simulink model "out_stage_test"  (R2020a)
settings: Solver=VariableStepAuto  StartTime=0.0  StopTime=0.025  RelTol=1e-3
undefined symbols (not defined in the file): debouncer_cycles, FPGA_CLK, FPGA_Ts, MECOS_CTRLR_Ts, PHCTRLR_CLK
libraries: xbsIndex_r4 x55, simulink x1
settings Model: Creator=valbas  LastModifiedBy=valbas

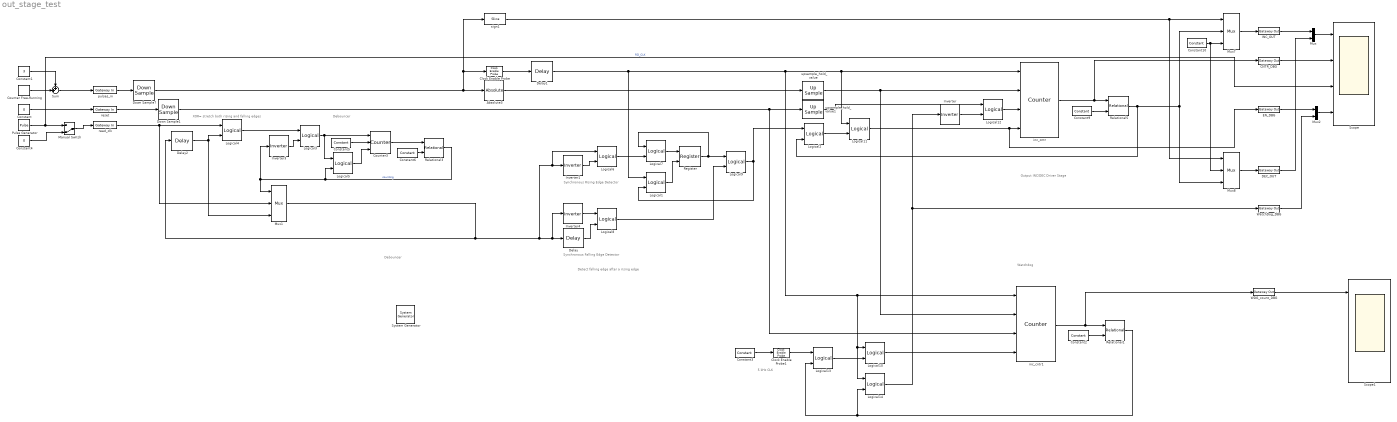
== system out_stage_test ==
  note: Output INC/DEC Driver Stage
  note: XOR= stretch both rising and falling edges
  note: Debouncer
  note: Synchronous Rising Edge Detector
  note: Synchronous Falling Edge Detector
  note: Debouncer
  note: Detect falling edge after a rising edge
  note: Watchdog
  note: 5 kHz CLK
  " System Generator" : xbsIndex_r4/ System Generator  Tag=genX  xilinxfamily=zynquplus  part=xczu7ev  speed=-2-e  package=ffvc1156  synthesis_tool=Vivado  clock_wrapper=Clock Enables  directory=./netlist  proj_type=Vivado  Synth_file=Vivado Synthesis Defaults  Impl_file=Vivado Implementation Defaults  testbench=off  simulink_period=FPGA_Ts  sysclk_period=FPGA_Ts*1e9  dcm_input_clock_period=10  incr_netlist=off  trim_vbits=Everywhere in SubSystem  dbl_ovrd=According to Block Masks  core_generation=According to Block Masks  run_coregen=off  deprecated_control=off  eval_field=0  block_type=sysgen
  Absolute3 : xbsIndex_r4/Absolute  precision=User Defined  arith_type="Signed  (2's comp)"  n_bits=22  bin_pt=0  quantization=Truncate  overflow=Wrap  en=off  latency=0  dbl_ovrd=off  block_type=abs
  CNTR_DBG : xbsIndex_r4/Gateway Out  inherit_from_input=on  hdl_port=on  rows=1  columns=1  UseAsDAC=off  DACChannel='1'  interface=None  automatic_assignment=on  address_offset=hex2dec('00')  intf_name=''  intf_description=''  timing_constraint=None  locs_specified=off  LOCs={}  io_standard={}  block_type=gatewayout
  Clock Enable Probe : xbsIndex_r4/Clock Enable Probe  inherit_constraints=on  block_type=ceprobe
      settings: infoedit="Clock enable extractor.  Produces a Boolean output that mirrors the hardware clock enable associated with the input sample rate.<br><br>Hardware notes: in hardware this block costs nothing."
  Clock Enable Probe1 : xbsIndex_r4/Clock Enable Probe  inherit_constraints=on  block_type=ceprobe
      settings: infoedit="Clock enable extractor.  Produces a Boolean output that mirrors the hardware clock enable associated with the input sample rate.<br><br>Hardware notes: in hardware this block costs nothing."
  Constant : Constant  Value=0
  Constant1 : Constant  Value=3
  Constant10 : xbsIndex_r4/Constant  const=0  gui_display_data_type=Boolean  arith_type=Boolean  n_bits=22  bin_pt=0  preci_type=Single  exp_width=8  frac_width=24  explicit_period=off  period=1  equ=P=C  opselect=C  inp2=PCIN>>17  opr=+  inp1=P  carry=CIN  dbl_ovrd=off  block_type=constant
  Constant2 : xbsIndex_r4/Constant  const=0  gui_display_data_type=Fixed-point  arith_type=Signed (2's comp)  n_bits=22  bin_pt=0  preci_type=Single  exp_width=8  frac_width=24  explicit_period=off  period=1  equ=P=C  opselect=C  inp2=PCIN>>17  opr=+  inp1=P  carry=CIN  dbl_ovrd=off  block_type=constant
  Constant3 : xbsIndex_r4/Constant  const=1  gui_display_data_type=Boolean  arith_type=Boolean  n_bits=7  bin_pt=0  preci_type=Single  exp_width=8  frac_width=24  explicit_period=on  period=PWM_Ts  equ=P=C  opselect=C  inp2=PCIN>>17  opr=+  inp1=P  carry=CIN  dbl_ovrd=off  block_type=constant
  Constant4 : Constant  Value=0
  Constant5 : xbsIndex_r4/Constant  const=debouncer_cycles  gui_display_data_type=Fixed-point  arith_type=Unsigned  n_bits=7  bin_pt=0  preci_type=Single  exp_width=8  frac_width=24  explicit_period=off  period=1  equ=P=C  opselect=C  inp2=PCIN>>17  opr=+  inp1=P  carry=CIN  dbl_ovrd=off  block_type=constant
  Constant6 : xbsIndex_r4/Constant  const=1  gui_display_data_type=Fixed-point  arith_type=Unsigned  n_bits=7  bin_pt=0  preci_type=Single  exp_width=8  frac_width=24  explicit_period=off  period=1  equ=P=C  opselect=C  inp2=PCIN>>17  opr=+  inp1=P  carry=CIN  dbl_ovrd=off  block_type=constant
  Constant9 : xbsIndex_r4/Constant  const=0  gui_display_data_type=Fixed-point  arith_type=Signed (2's comp)  n_bits=22  bin_pt=0  preci_type=Single  exp_width=8  frac_width=24  explicit_period=off  period=1  equ=P=C  opselect=C  inp2=PCIN>>17  opr=+  inp1=P  carry=CIN  dbl_ovrd=off  block_type=constant
  Counter Free-Running : simulink/Sources/Counter Free-Running  NumBits=4  tsamp=PHCTRLR_Ts
  Counter3 : xbsIndex_r4/Counter  cnt_type=Free Running  cnt_to=2  operation=Down  start_count=1  cnt_by_val=1  arith_type=Unsigned  n_bits=7  bin_pt=0  load_pin=on  rst=off  en=on  explicit_period=on  period=FPGA_Ts  use_behavioral_HDL=off  implementation=Fabric  dbl_ovrd=off  block_type=counter
  DEC_OUT : xbsIndex_r4/Gateway Out  inherit_from_input=on  hdl_port=on  rows=1  columns=1  UseAsDAC=off  DACChannel='1'  interface=None  automatic_assignment=on  address_offset=hex2dec('00')  intf_name=''  intf_description=''  timing_constraint=None  locs_specified=off  LOCs={}  io_standard={}  block_type=gatewayout
  Delay : xbsIndex_r4/Delay  rst=off  infoeditControl=Selection of Reset will increase slice count due to use of real FFs and instead of SRLs  en=off  latency=1  reg_retiming=off  dbl_ovrd=off  block_type=delay
  Delay1 : xbsIndex_r4/Delay  rst=off  infoeditControl=Selection of Reset will increase slice count due to use of real FFs and instead of SRLs  en=off  latency=1  reg_retiming=off  dbl_ovrd=off  block_type=delay
  Delay2 : xbsIndex_r4/Delay  rst=off  infoeditControl=Selection of Reset will increase slice count due to use of real FFs and instead of SRLs  en=off  latency=1  reg_retiming=off  dbl_ovrd=off  block_type=delay
  Down Sample1 : xbsIndex_r4/Down Sample  sample_ratio=FPGA_CLK/PHCTRLR_CLK  sample_phase="Last Value of Frame  (most efficient)"  en=off  rst=off  latency=1  dbl_ovrd=off  block_type=dsamp
  Down Sample7 : xbsIndex_r4/Down Sample  sample_ratio=FPGA_CLK/PHCTRLR_CLK  sample_phase="Last Value of Frame  (most efficient)"  en=off  rst=off  latency=1  dbl_ovrd=off  block_type=dsamp
  EN_DBG : xbsIndex_r4/Gateway Out  inherit_from_input=on  hdl_port=on  rows=1  columns=1  UseAsDAC=off  DACChannel='1'  interface=None  automatic_assignment=on  address_offset=hex2dec('00')  intf_name=''  intf_description=''  timing_constraint=None  locs_specified=off  LOCs={}  io_standard={}  block_type=gatewayout
  INC_OUT : xbsIndex_r4/Gateway Out  inherit_from_input=on  hdl_port=on  rows=1  columns=1  UseAsDAC=off  DACChannel='1'  interface=None  automatic_assignment=on  address_offset=hex2dec('00')  intf_name=''  intf_description=''  timing_constraint=None  locs_specified=off  LOCs={}  io_standard={}  block_type=gatewayout
  Inverter : xbsIndex_r4/Inverter  en=off  latency=0  dbl_ovrd=off  block_type=inv
  Inverter1 : xbsIndex_r4/Inverter  en=off  latency=1  dbl_ovrd=off  block_type=inv
  Inverter3 : xbsIndex_r4/Inverter  en=off  latency=0  dbl_ovrd=off  block_type=inv
  Inverter4 : xbsIndex_r4/Inverter  en=off  latency=0  dbl_ovrd=off  block_type=inv
  Logical{1,5,7,10..12,14} (7 alike) : xbsIndex_r4/Logical  logical_function=OR  inputs=2  en=off  latency=0  precision=Full  arith_type=Unsigned  n_bits=16  bin_pt=0  align_bp=on  dbl_ovrd=off  block_type=logical
  Logical{2..3,6,8..9,13} (6 alike) : xbsIndex_r4/Logical  logical_function=AND  inputs=2  en=off  latency=0  precision=Full  arith_type=Unsigned  n_bits=16  bin_pt=0  align_bp=on  dbl_ovrd=off  block_type=logical
  Logical4 : xbsIndex_r4/Logical  logical_function=XOR  inputs=2  en=off  latency=0  precision=Full  arith_type=Unsigned  n_bits=16  bin_pt=0  align_bp=on  dbl_ovrd=off  block_type=logical
  Manual Switch : ManualSwitch  CurrentSetting=0
  Mux : Mux  Inputs=2
  Mux1 : xbsIndex_r4/Mux  inputs=2  en=off  latency=0  precision=Full  arith_type=Unsigned  n_bits=16  bin_pt=14  quantization=Truncate  overflow=Wrap  dbl_ovrd=off  block_type=mux
  Mux2 : Mux  Inputs=2
  Mux7 : xbsIndex_r4/Mux  inputs=2  en=off  latency=0  precision=Full  arith_type=Unsigned  n_bits=16  bin_pt=14  quantization=Truncate  overflow=Wrap  dbl_ovrd=off  block_type=mux
  Mux8 : xbsIndex_r4/Mux  inputs=2  en=off  latency=0  precision=Full  arith_type=Unsigned  n_bits=16  bin_pt=14  quantization=Truncate  overflow=Wrap  dbl_ovrd=off  block_type=mux
  Pulse Generator : DiscretePulseGenerator  PulseType=Time based  Period=MECOS_CTRLR_Ts  PulseWidth=50
  Register : xbsIndex_r4/Register  init=0  rst=on  en=off  dbl_ovrd=off  block_type=register
  Relational1 : xbsIndex_r4/Relational  mode=a!=b  op_type=Bool  en=off  latency=0  dbl_ovrd=off  block_type=relational
  Relational3 : xbsIndex_r4/Relational  mode=a!=b  op_type=Bool  en=off  latency=0  dbl_ovrd=off  block_type=relational
  Relational5 : xbsIndex_r4/Relational  mode=a!=b  op_type=Bool  en=off  latency=0  dbl_ovrd=off  block_type=relational
  Scope : Scope  NumInputPorts=4
  Scope1 : Scope  NumInputPorts=4
  Sum : Sum  Inputs=++|
  WDG_count_DBG : xbsIndex_r4/Gateway Out  inherit_from_input=on  hdl_port=on  rows=1  columns=1  UseAsDAC=off  DACChannel='1'  interface=None  automatic_assignment=on  address_offset=hex2dec('00')  intf_name=''  intf_description=''  timing_constraint=None  locs_specified=off  LOCs={}  io_standard={}  block_type=gatewayout
  WatchDog_DBG : xbsIndex_r4/Gateway Out  inherit_from_input=on  hdl_port=on  rows=1  columns=1  UseAsDAC=off  DACChannel='1'  interface=None  automatic_assignment=on  address_offset=hex2dec('00')  intf_name=''  intf_description=''  timing_constraint=None  locs_specified=off  LOCs={}  io_standard={}  block_type=gatewayout
  inc_cntr : xbsIndex_r4/Counter  cnt_type=Free Running  cnt_to=0  operation=Down  start_count=0  cnt_by_val=1  arith_type="Signed  (2's comp)"  n_bits=22  bin_pt=0  load_pin=on  rst=on  en=on  explicit_period=on  period=FPGA_Ts  use_behavioral_HDL=off  implementation=DSP48  dbl_ovrd=off  block_type=counter
  inc_cntr1 : xbsIndex_r4/Counter  cnt_type=Free Running  cnt_to=0  operation=Down  start_count=0  cnt_by_val=1  arith_type="Signed  (2's comp)"  n_bits=22  bin_pt=0  load_pin=on  rst=on  en=on  explicit_period=on  period=FPGA_Ts  use_behavioral_HDL=off  implementation=DSP48  dbl_ovrd=off  block_type=counter
  pulses_in : xbsIndex_r4/Gateway In  gui_display_data_type=Fixed-point  arith_type="Signed  (2's comp)"  n_bits=22  bin_pt=0  preci_type=Single  exp_width=8  frac_width=24  rows=1  columns=1  quantization="Round  (unbiased: +/- Inf)"  overflow=Saturate  period=FPGA_Ts  UseAsADC=off  ADCChannel='1'  interface=None  automatic_assignment=on  address_offset=hex2dec('00')  intf_name=''  intf_description=''  default_value=0  timing_constraint=None  locs_specified=off  LOCs={}  io_standard={}  inherit_from_input=off  hdl_port=on  dbl_ovrd=off  block_type=gatewayin
  read_clk : xbsIndex_r4/Gateway In  gui_display_data_type=Boolean  arith_type=Boolean  n_bits=16  bin_pt=14  preci_type=Single  exp_width=8  frac_width=24  rows=1  columns=1  quantization="Round  (unbiased: +/- Inf)"  overflow=Saturate  period=FPGA_Ts  UseAsADC=off  ADCChannel='1'  interface=None  automatic_assignment=on  address_offset=hex2dec('00')  intf_name=''  intf_description=''  default_value=0  timing_constraint=None  locs_specified=off  LOCs={}  io_standard={}  inherit_from_input=off  hdl_port=on  dbl_ovrd=off  block_type=gatewayin
  reset : xbsIndex_r4/Gateway In  gui_display_data_type=Boolean  arith_type=Boolean  n_bits=16  bin_pt=14  preci_type=Single  exp_width=8  frac_width=24  rows=1  columns=1  quantization="Round  (unbiased: +/- Inf)"  overflow=Saturate  period=FPGA_Ts  UseAsADC=off  ADCChannel='1'  interface=None  automatic_assignment=on  address_offset=hex2dec('00')  intf_name=''  intf_description=''  default_value=0  timing_constraint=None  locs_specified=off  LOCs={}  io_standard={}  inherit_from_input=off  hdl_port=on  dbl_ovrd=off  block_type=gatewayin
  sign1 : xbsIndex_r4/Slice  nbits=1  boolean_output=on  mode=Upper Bit Location + Width  bit1=0  base1=MSB of Input  bit0=0  base0=LSB of Input  dbl_ovrd=off  block_type=slice
  upsample_hold_value : xbsIndex_r4/Up Sample  sample_ratio=FPGA_CLK/PHCTRLR_CLK  copy_samples=on  en=off  latency=0  dbl_ovrd=off  block_type=usamp
  upsample_hold_value1 : xbsIndex_r4/Up Sample  sample_ratio=FPGA_CLK/PHCTRLR_CLK  copy_samples=on  en=off  latency=0  dbl_ovrd=off  block_type=usamp
  wires:
  Delay1/1 -> Logical1/1, Logical14/1, Logical10/1, inc_cntr1/1, inc_cntr/1, Logical11/1
  Mux7/1 -> INC_OUT/1
  Constant9/1 -> Relational5/2
  Relational5/1 -> Logical2/2, Mux8/3, Mux7/2
  inc_cntr/1 -> CNTR_DBG/1, Relational5/1
  Down Sample7/1 -> sign1/1, Clock Enable Probe/1, Absolute3/1
  Constant10/1 -> Mux8/2, Mux7/3
  sign1/1 -> Mux8/1, Mux7/1
  Mux8/1 -> DEC_OUT/1
  Down Sample1/1 -> inc_cntr1/3, upsample_hold_value1/1
  Logical11/1 -> EN_DBG/1, inc_cntr/4
  upsample_hold_value/1 -> inc_cntr1/2, inc_cntr/2
  Logical2/1 -> Logical11/2
  Constant/1 -> reset/1
  Pulse Generator/1 -> Manual Switch/1, Scope/3  "RD_CLK"
  Counter Free-Running/1 -> Sum/2
  Sum/1 -> pulses_in/1
  Constant1/1 -> Sum/1
  INC_OUT/1 -> Mux/1
  DEC_OUT/1 -> Mux/2
  Mux/1 -> Scope/1
  CNTR_DBG/1 -> Scope/2
  EN_DBG/1 -> Mux2/1
  Logical5/1 -> Counter3/3
  Counter3/1 -> Relational3/1
  Delay2/1 -> Mux1/3, Logical4/2
  Logical4/1 -> Logical3/1
  Logical3/1 -> Logical5/1, Counter3/1
  Constant5/1 -> Counter3/2
  Relational3/1 -> Mux1/1, Inverter3/1, Logical5/2  "counting"
  Inverter3/1 -> Logical3/2
  read_clk/1 -> Logical4/1, Mux1/2
  Constant6/1 -> Relational3/2
  Logical6/1 -> Logical7/2
  Inverter1/1 -> Logical6/2
  Logical7/1 -> Register/1
  Register/1 -> Logical9/1, Logical7/1
  Inverter4/1 -> Logical8/1
  Mux1/1 -> Delay2/1, Logical6/1, Inverter1/1, Inverter4/1, Delay/1
  Delay/1 -> Logical8/2
  Logical8/1 -> Logical9/2
  Logical9/1 -> Logical1/2, Logical2/1
  Logical1/1 -> Register/2
  Constant2/1 -> Relational1/2
  Absolute3/1 -> upsample_hold_value/1
  Relational1/1 -> Logical14/2, Logical13/2
  inc_cntr1/1 -> WDG_count_DBG/1, Relational1/1
  Logical12/1 -> inc_cntr/3
  upsample_hold_value1/1 -> Logical12/1
  Mux2/1 -> Scope/4
  WatchDog_DBG/1 -> Mux2/2
  reset/1 -> Down Sample1/1
  pulses_in/1 -> Down Sample7/1
  Inverter/1 -> Logical12/2
  WDG_count_DBG/1 -> Scope1/1
  Constant3/1 -> Clock Enable Probe1/1
  Clock Enable Probe1/1 -> Logical13/1
  Clock Enable Probe/1 -> Delay1/1
  Logical13/1 -> Logical10/2
  Logical10/1 -> inc_cntr1/4
  Logical14/1 -> WatchDog_DBG/1, Inverter/1
  Constant4/1 -> Manual Switch/2
  Manual Switch/1 -> read_clk/1
